simulink model "dynamic_model"  (R2021a)
settings: Solver=ode4  StartTime=0.0  StopTime=1  FixedStep=0.001  RelTol=1e-3
libraries: slpidlib x2
settings Model: Creator=Samuel  LastModifiedBy=Samuel

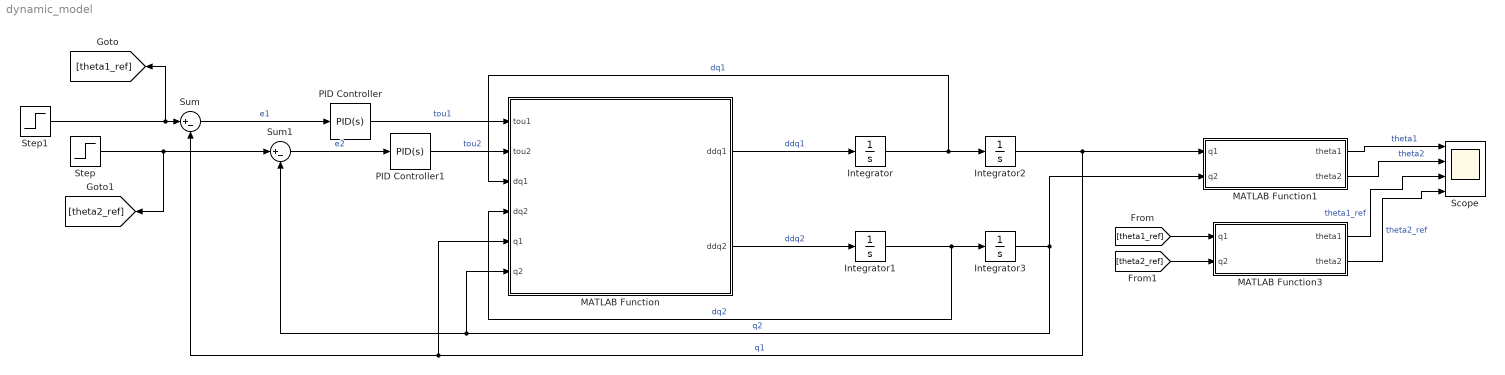
== system dynamic_model ==
  Integrator{,1..3} (4 alike) : Integrator
  MATLAB Function : MATLAB Function  TreatAsAtomicUnit=on
  MATLAB Function1 : MATLAB Function  TreatAsAtomicUnit=on
  MATLAB Function3 : MATLAB Function  TreatAsAtomicUnit=on
  PID Controller : slpidlib/PID Controller  Controller=PID  Form=Parallel  TimeDomain=Continuous-time  UseExternalTs=off  SampleTime=-1  IntegratorMethod=Forward Euler  FilterMethod=Forward Euler  ControllerParametersSource=internal  P=37.3891280078924  I=7.71354505395236  D=4.87996499047848  UseFilter=on  N=2771.20189567062  TunerSelectOption=Transfer Function Based (PID Tuner App)  InitialConditionSource=internal  InitialConditionForIntegrator=0  InitialConditionForFilter=0  DifferentiatorICPrevScaledInput=0  ExternalReset=none  TrackingMode=off  Kt=1  LimitOutput=off  SatLimitsSource=internal  UpperSaturationLimit=inf  LowerSaturationLimit=-inf  LinearizeAsGain=on  AntiWindupMode=none  Kb=1  POutMin=[]  POutMax=[]  IOutMin=[]  IOutMax=[]  DOutMin=[]  DOutMax=[]  NOutMin=[]  NOutMax=[]  SumOutMin=[]  SumOutMax=[]  SaturationOutMin=[]  SaturationOutMax=[]  PParamMin=[]  PParamMax=[]  IParamMin=[]  IParamMax=[]  DParamMin=[]  DParamMax=[]  NParamMin=[]  NParamMax=[]  KbParamMin=[]  KbParamMax=[]  KtParamMin=[]  KtParamMax=[]  KbOutMin=[]  KbOutMax=[]  KtOutMin=[]  KtOutMax=[]  IntegratorOutMin=[]  IntegratorOutMax=[]  FilterOutMin=[]  FilterOutMax=[]  SumI1OutMin=[]  SumI1OutMax=[]  SumI2OutMin=[]  SumI2OutMax=[]  SumI3OutMin=[]  SumI3OutMax=[]  SumI4OutMin=[]  SumI4OutMax=[]  SumDOutMin=[]  SumDOutMax=[]  DifferentiatorOutMin=[]  DifferentiatorOutMax=[]  FilterDiffOutCoefMin=[]  FilterDiffOutCoefMax=[]  ReciprocalOutMin=[]  ReciprocalOutMax=[]  SumDenOutMin=[]  SumDenOutMax=[]  SumNumOutMin=[]  SumNumOutMax=[]  DivideOutMin=[]  DivideOutMax=[]  UdiffTsProdOutMin=[]  UdiffTsProdOutMax=[]  NTsProdOutMin=[]  NTsProdOutMax=[]  UintegralTsProdOutMin=[]  UintegralTsProdOutMax=[]  UngainTsProdOutMin=[]  UngainTsProdOutMax=[]  IntegratorContinuousStateAttributes=''  IntegratorStateMustResolveToSignalObject=off  IntegratorRTWStateStorageClass=Auto  FilterContinuousStateAttributes=''  FilterStateMustResolveToSignalObject=off  FilterRTWStateStorageClass=Auto  ParallelPVariant=InternalParameters  IdealPVariant=Disabled  IVariant=InternalParameters  DVariant=InternalParameters  IntegratorVariant=Continuous  SatVariant=Disabled  AWVariant=Passthrough  PCopyVariant=Disabled  TRVariant=Disabled  FdbkBlocksVariant=Forward  IdealPFdbkVariant=Disabled  SatFdbkVariant=Disabled  DerivativeFilterVariant=ContFilter  NVariant=InternalParameters  NCopyVariant=Disabled  FilterICVariant=InternalICsFilter  IntegratorICVariant=InternalICs  ExternalResetVariant=Disabled  TRSumVariant=Passthrough  SumFdbkVariant=Disabled  SumVariant=Sum_PID  TsampFilterVariant=InternalTs  TsampNgainVariant=Passthrough  TsampIntegralVariant=Passthrough  ExternalSaturationOutDataTypeStr=Inherit: Same as second input
  PID Controller1 : slpidlib/PID Controller  Controller=PID  Form=Parallel  TimeDomain=Continuous-time  UseExternalTs=off  SampleTime=-1  IntegratorMethod=Forward Euler  FilterMethod=Forward Euler  ControllerParametersSource=internal  P=376.159220848573  I=13257.1508691485  D=2.39862827753367  UseFilter=on  N=2849.45170110993  TunerSelectOption=Transfer Function Based (PID Tuner App)  InitialConditionSource=internal  InitialConditionForIntegrator=0  InitialConditionForFilter=0  DifferentiatorICPrevScaledInput=0  ExternalReset=none  TrackingMode=off  Kt=1  LimitOutput=off  SatLimitsSource=internal  UpperSaturationLimit=inf  LowerSaturationLimit=-inf  LinearizeAsGain=on  AntiWindupMode=none  Kb=1  POutMin=[]  POutMax=[]  IOutMin=[]  IOutMax=[]  DOutMin=[]  DOutMax=[]  NOutMin=[]  NOutMax=[]  SumOutMin=[]  SumOutMax=[]  SaturationOutMin=[]  SaturationOutMax=[]  PParamMin=[]  PParamMax=[]  IParamMin=[]  IParamMax=[]  DParamMin=[]  DParamMax=[]  NParamMin=[]  NParamMax=[]  KbParamMin=[]  KbParamMax=[]  KtParamMin=[]  KtParamMax=[]  KbOutMin=[]  KbOutMax=[]  KtOutMin=[]  KtOutMax=[]  IntegratorOutMin=[]  IntegratorOutMax=[]  FilterOutMin=[]  FilterOutMax=[]  SumI1OutMin=[]  SumI1OutMax=[]  SumI2OutMin=[]  SumI2OutMax=[]  SumI3OutMin=[]  SumI3OutMax=[]  SumI4OutMin=[]  SumI4OutMax=[]  SumDOutMin=[]  SumDOutMax=[]  DifferentiatorOutMin=[]  DifferentiatorOutMax=[]  FilterDiffOutCoefMin=[]  FilterDiffOutCoefMax=[]  ReciprocalOutMin=[]  ReciprocalOutMax=[]  SumDenOutMin=[]  SumDenOutMax=[]  SumNumOutMin=[]  SumNumOutMax=[]  DivideOutMin=[]  DivideOutMax=[]  UdiffTsProdOutMin=[]  UdiffTsProdOutMax=[]  NTsProdOutMin=[]  NTsProdOutMax=[]  UintegralTsProdOutMin=[]  UintegralTsProdOutMax=[]  UngainTsProdOutMin=[]  UngainTsProdOutMax=[]  IntegratorContinuousStateAttributes=''  IntegratorStateMustResolveToSignalObject=off  IntegratorRTWStateStorageClass=Auto  FilterContinuousStateAttributes=''  FilterStateMustResolveToSignalObject=off  FilterRTWStateStorageClass=Auto  ParallelPVariant=InternalParameters  IdealPVariant=Disabled  IVariant=InternalParameters  DVariant=InternalParameters  IntegratorVariant=Continuous  SatVariant=Disabled  AWVariant=Passthrough  PCopyVariant=Disabled  TRVariant=Disabled  FdbkBlocksVariant=Forward  IdealPFdbkVariant=Disabled  SatFdbkVariant=Disabled  DerivativeFilterVariant=ContFilter  NVariant=InternalParameters  NCopyVariant=Disabled  FilterICVariant=InternalICsFilter  IntegratorICVariant=InternalICs  ExternalResetVariant=Disabled  TRSumVariant=Passthrough  SumFdbkVariant=Disabled  SumVariant=Sum_PID  TsampFilterVariant=InternalTs  TsampNgainVariant=Passthrough  TsampIntegralVariant=Passthrough  ExternalSaturationOutDataTypeStr=Inherit: Same as second input
  Scope : Scope  NumInputPorts=4
  Step : Step  Time=0  After=pi/10  SampleTime=0
  Step1 : Step  Time=0  After=pi/18  SampleTime=0
  Sum : Sum  Inputs=|+-
  Sum1 : Sum  Inputs=|+-
  wires:
  MATLAB Function/2(ddq2) -> Integrator1/1  "ddq2"
  MATLAB Function/1(ddq1) -> Integrator/1  "ddq1"
  Integrator/1 -> MATLAB Function/3(dq1), Integrator2/1  "dq1"
  Integrator1/1 -> Integrator3/1, MATLAB Function/4(dq2)  "dq2"
  Sum/1 -> PID Controller/1  "e1"
  Sum1/1 -> PID Controller1/1  "e2"
  PID Controller/1 -> MATLAB Function/1(tou1)  "tou1"
  PID Controller1/1 -> MATLAB Function/2(tou2)  "tou2"
  Step1/1 -> [theta1_ref], Sum/1
  Step/1 -> Sum1/1, [theta2_ref]
  MATLAB Function1/1(theta1) -> Scope/1  "theta1"
  MATLAB Function1/2(theta2) -> Scope/2  "theta2"
  Integrator3/1 -> Sum1/2, MATLAB Function/6(q2), MATLAB Function1/2(q2)  "q2"
  Integrator2/1 -> MATLAB Function1/1(q1), MATLAB Function/5(q1), Sum/2  "q1"
  [theta1_ref] -> MATLAB Function3/1(q1)
  [theta2_ref] -> MATLAB Function3/2(q2)
  MATLAB Function3/1(theta1) -> Scope/3  "theta1_ref"
  MATLAB Function3/2(theta2) -> Scope/4  "theta2_ref"

== matlab function dynamic_model/MATLAB Function1 ==
  data: q1 input; theta1 output; q2 input; theta2 output
function [theta1, theta2] = rad2deg(q1,q2)

theta1 = rad2deg(q1);
theta2 = rad2deg(q2);

== matlab function dynamic_model/MATLAB Function ==
  data: tou1 input; ddq1 output; tou2 input; ddq2 output; dq1 input; dq2 input; q1 input; q2 input
function [ddq1,ddq2] = Dynamic_model(tou1, tou2,dq1, dq2,q1,q2)
    m1 = 0.1;%(kg)
    m2 = 0.1;%(kg)
    l1 = 0.8;%(m)
    l2 = 0.4;%(m)
    g = 9.81;%m/s^2
    
    c1 = cos(q1);
    c2 = cos(q2);
    s1 = sin(q1);
    s2 = sin(q2);
    
    c12 = cos(q1+q2);
    s12 = sin(q1+q2);
    
    M = [(m1 + m2)*l1*l1 + m2*l2*l2 + 2*m2*l1*l2*c2,   m2*l2*l2 + m2*l1*l2*c2;
                    m2*l2*l2 + m2*l1*l2*c2,                         m2*l2*l2];
                
    C = [-2*m2*l1*l2*s2*dq1*dq2 - m2*l1*l2*s2*dq2*dq2;
                             m2*l1*l2*c2*dq1*dq1];

    G = [(m1+m2)*g*l1*c1 + m2*g*l2*c12;
                                m2*g*l1*c12];
    torque = [tou1;
              tou2];
    
    
                            
    %ddq = M\(torque - C- G);
    ddq = M\(torque -C-G);
    ddq1 = ddq(1);
    ddq2 = ddq(2);
    M1=M(1,1);
    M2 = M(1,2);
    M3 = M(2,1);
    M4 = M(2,2);

== matlab function dynamic_model/MATLAB Function3 ==
  data: q1 input; theta1 output; q2 input; theta2 output
function [theta1, theta2] = rad2deg(q1,q2)

theta1 = rad2deg(q1);
theta2 = rad2deg(q2);
